simulink model "Model_120S2P"  (R2019b)
settings: Solver=VariableStepAuto  StartTime=0.0  StopTime=800  RelTol=1e-3
libraries: fl_lib x29, nesl_utility x6, simulink x2, hwlogiciolib x1, ee_lib x1
(part 1 of 3)
settings Model: SimulationMode=accelerator  Creator=ZHOU Jinhan  LastModifiedBy=ZHOU Jinhan

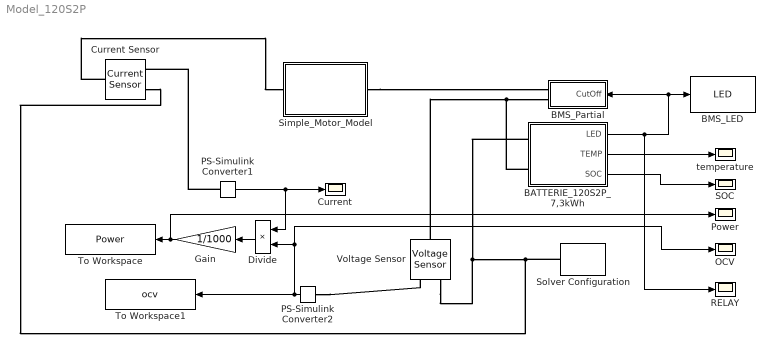
== system Model_120S2P ==
  BATTERIE_120S2P_7,3kWh : Subsystem
  BMS_LED : hwlogiciolib/LED  NumLeds=1  LastTargetBoard=None
      settings: SourceProductName=SoC Blockset  SourceProductBaseCode=HW
  BMS_Partial : Subsystem
  Current : Scope
  Current Sensor : fl_lib/Electrical/Electrical Sensors/Current Sensor
  Divide : Product  Inputs=**
  Gain : Gain  Gain=1/1000
  OCV : Scope
  PS-Simulink Converter1 : nesl_utility/PS-Simulink Converter  PhysicalDomain=network_engine_domain  SubClassName=ps_output  LeftPortType=input  RightPortType=output  PseudoPeriodic=off  Frequencies=[]  Unit=inherit  AffineConversion=off
  PS-Simulink Converter2 : nesl_utility/PS-Simulink Converter  PhysicalDomain=network_engine_domain  SubClassName=ps_output  LeftPortType=input  RightPortType=output  PseudoPeriodic=off  Frequencies=[]  Unit=inherit  AffineConversion=off
  Power : Scope
  RELAY : Scope
  SOC : Scope
  Simple_Motor_Model : Subsystem
  Solver Configuration : nesl_utility/Solver Configuration  PhysicalDomain=network_engine_domain  SubClassName=solver  LeftPortType=input  RightPortType=generic  Tones=[]  Harmonics=[]  SimulateNoise=off  Profile=off  UseLocalSampling=off  EnableSwitchedLinearOptims=on  FrequencyDomain=off  UseCCode=off  RelTol=0.001  AbsTol=1e-06  MinStep=1e-09  ToWorkspace=off  RevertToSquareIcSolve=off  NumHomotopyIterations=100  PhasorMode=off  PhasorModeNumHarmonics=1  DoDC=off  ResidualTolerance=1e-09  UseLocalSolver=on  LocalSolverChoice=NE_BACKWARD_EULER_ADVANCER  LocalSolverSampleTime=0.2  DoFixedCost=on  MaxNonlinIter=3  MaxModeIter=2  LinearAlgebra=auto  EquationFormulation=NE_TIME_EF  DelaysMemoryBudget=1024  AutomaticFiltering=on  FilteringTimeConstant=0.001  PartitionStorageMethod=AS_NEEDED  PartitionMemoryBudget=1024  PartitionMethod=ROBUST
  To Workspace : ToWorkspace  VariableName=Power  SaveFormat=Timeseries  SampleTime=-1
  To Workspace1 : ToWorkspace  VariableName=ocv  SaveFormat=Timeseries  SampleTime=-1
  Voltage Sensor : fl_lib/Electrical/Electrical Sensors/Voltage Sensor
  temperature : Scope
  wires:
  BATTERIE_120S2P_7,3kWh/3(SOC) -> SOC/1
  PS-Simulink Converter2/1 -> Divide/2, OCV/1, To Workspace1/1
  Divide/1 -> Gain/1
  BATTERIE_120S2P_7,3kWh/2(TEMP) -> temperature/1
  Gain/1 -> Power/1, To Workspace/1
  BATTERIE_120S2P_7,3kWh/1(LED) -> RELAY/1, BMS_Partial/1(CutOff), BMS_LED/1
  PS-Simulink Converter1/1 -> Current/1, Divide/1
  connections:
  PS-Simulink Converter1/LConn1 -- Current Sensor/RConn1
  BATTERIE_120S2P_7,3kWh/LConn1 -- Voltage Sensor/RConn2 -- Current Sensor/RConn2 -- Solver Configuration/RConn1
  PS-Simulink Converter2/LConn1 -- Voltage Sensor/RConn1
  Simple_Motor_Model/RConn1 -- BMS_Partial/RConn1
  BATTERIE_120S2P_7,3kWh/LConn2 -- Voltage Sensor/LConn1 -- BMS_Partial/RConn2
  Current Sensor/LConn1 -- Simple_Motor_Model/LConn1
